simulink model "car_dynamics_sim"  (R2019b)
settings: Solver=VariableStepAuto  StartTime=0.0  StopTime=100  RelTol=1e-3
values from neighbouring files (symbols this model uses):
  air_density = 1.225    [main.m]
  drag_coefficient = 0.33    [main.m]
  equ_mass_of_rot_parts = (1/wheel_radius^2)*(wheel_inertia+motor_rotor_inertia*gearbox_ratio^2)    (= 15.059687787)    [main.m]
  gravity = 9.8    [main.m]
  mass = 900    [main.m]
  rolling_resistance_coefficient_0 = 0    [main.m]
  rolling_resistance_coefficient_1 = 0.01    [main.m]
  slope_of_track = 3    [main.m]
  surface_area = 2.14    [main.m]
  torque = 150    [main.m]
  wheel_radius = 0.165    [main.m]
undefined symbols (not defined in the file or in its folder): simulation_length_track
settings Model: Creator=jamil  LastModifiedBy=jamil

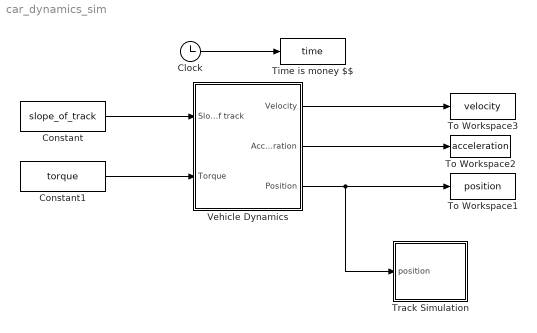
== system car_dynamics_sim ==
  Clock : Clock
  Constant : Constant  Value=slope_of_track
  Constant1 : Constant  Value=torque
  Time is money $$ : ToWorkspace  VariableName=time  SampleTime=-1
  To Workspace1 : ToWorkspace  VariableName=position  SampleTime=-1
  To Workspace2 : ToWorkspace  VariableName=acceleration  SampleTime=-1
  To Workspace3 : ToWorkspace  VariableName=velocity  SampleTime=-1
  Track Simulation : Subsystem
  Vehicle Dynamics : Subsystem
  wires:
  Constant/1 -> Vehicle Dynamics/1("Slope of track ")
  Constant1/1 -> Vehicle Dynamics/2(Torque)
  Vehicle Dynamics/1(Velocity) -> To Workspace3/1
  Vehicle Dynamics/2(Acceleration) -> To Workspace2/1
  Clock/1 -> Time is money $$/1
  Vehicle Dynamics/3(Position) -> Track Simulation/1(position), To Workspace1/1

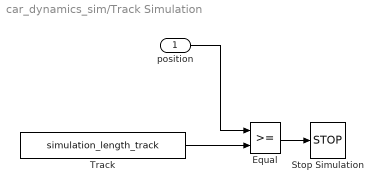
== system car_dynamics_sim/Track Simulation ==
  position : Inport
  Equal : RelationalOperator  OutDataTypeStr=boolean  RndMeth=Simplest
  Stop Simulation : Stop
  "Track " : Constant  Value=simulation_length_track
  wires:
  Equal/1 -> Stop Simulation/1
  position/1 -> Equal/1
  "Track "/1 -> Equal/2

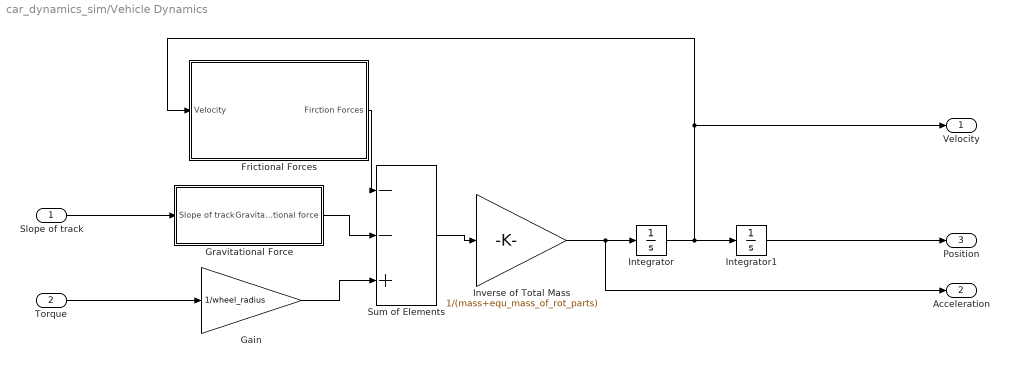
== system car_dynamics_sim/Vehicle Dynamics ==
  "Slope of track " : Inport
  Torque : Inport  Port=2
  Frictional Forces : Subsystem
  Gain : Gain  Gain=1/wheel_radius
  Gravitational Force : Subsystem
  Integrator : Integrator
  Integrator1 : Integrator
  Inverse of Total Mass : Gain  Gain=1/(mass+equ_mass_of_rot_parts)
  Sum of Elements : Sum  Inputs=--+
  Velocity : Outport
  Acceleration : Outport  Port=2
  Position : Outport  Port=3
  wires:
  Integrator/1 -> Integrator1/1, Frictional Forces/1(Velocity), Velocity/1
  Integrator1/1 -> Position/1
  Inverse of Total Mass/1 -> Acceleration/1, Integrator/1
  Sum of Elements/1 -> Inverse of Total Mass/1
  Frictional Forces/1(Firction Forces) -> Sum of Elements/1
  "Slope of track "/1 -> Gravitational Force/1(Slope of track)
  Gravitational Force/1(Gravitational force) -> Sum of Elements/2
  Torque/1 -> Gain/1
  Gain/1 -> Sum of Elements/3

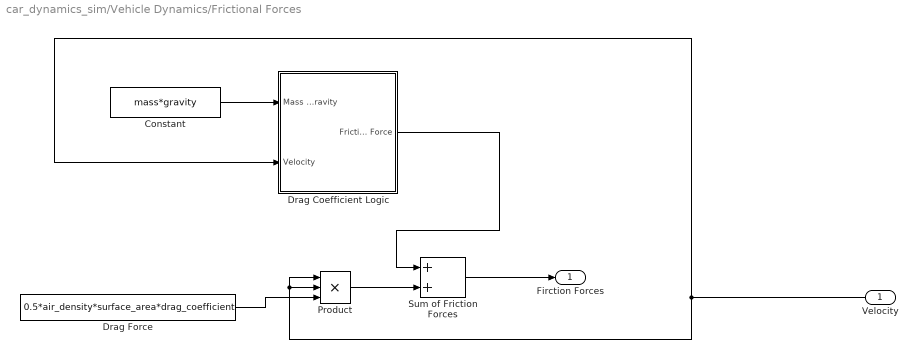
== system car_dynamics_sim/Vehicle Dynamics/Frictional Forces ==
  Velocity : Inport
  Constant : Constant  Value=mass*gravity
  Drag Coefficient Logic : Subsystem
  Drag Force : Constant  Value=0.5*air_density*surface_area*drag_coefficient
  Product : Product  Inputs=3
  Sum of Friction Forces : Sum
  Firction Forces : Outport
  wires:
  Sum of Friction Forces/1 -> Firction Forces/1
  Drag Force/1 -> Product/3
  Constant/1 -> Drag Coefficient Logic/1("Mass and Gravity ")
  Drag Coefficient Logic/1(Friction Force) -> Sum of Friction Forces/1
  Velocity/1 -> Drag Coefficient Logic/2(Velocity), Product/1, Product/2
  Product/1 -> Sum of Friction Forces/2

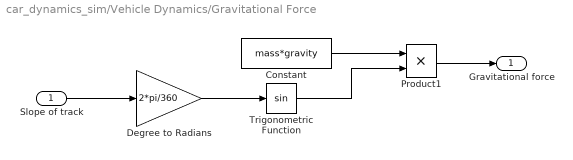
== system car_dynamics_sim/Vehicle Dynamics/Gravitational Force ==
  Slope of track : Inport
  Constant : Constant  Value=mass*gravity
  Degree to Radians : Gain  Gain=2*pi/360
  Product1 : Product
  Trigonometric Function : Trigonometry
  Gravitational force : Outport
  wires:
  Product1/1 -> Gravitational force/1
  Constant/1 -> Product1/1
  Trigonometric Function/1 -> Product1/2
  Slope of track/1 -> Degree to Radians/1
  Degree to Radians/1 -> Trigonometric Function/1

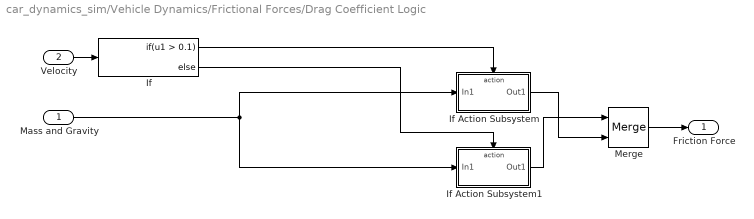
== system car_dynamics_sim/Vehicle Dynamics/Frictional Forces/Drag Coefficient Logic ==
  "Mass and Gravity " : Inport
  Velocity : Inport  Port=2
  If : If  IfExpression=u1 > 0.1
  If Action Subsystem : Subsystem  TreatAsAtomicUnit=on
  If Action Subsystem1 : Subsystem  TreatAsAtomicUnit=on
  Merge : Merge
  Friction Force : Outport
  wires:
  If Action Subsystem/1(Out1) -> Merge/2
  If Action Subsystem1/1(Out1) -> Merge/1
  If/2 -> If Action Subsystem1/Action
  "Mass and Gravity "/1 -> If Action Subsystem/1(In1), If Action Subsystem1/1(In1)
  Merge/1 -> Friction Force/1
  If/1 -> If Action Subsystem/Action
  Velocity/1 -> If/1

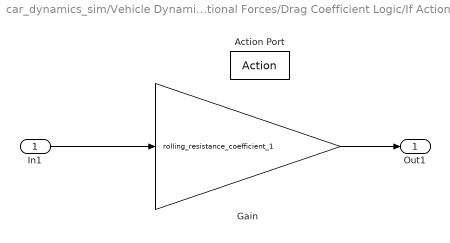
== system car_dynamics_sim/Vehicle Dynamics/Frictional Forces/Drag Coefficient Logic/If Action Subsystem ==
  In1 : Inport
  Action Port : ActionPort  ActionPortLabel=if(u1 > 0.1)
  Gain : Gain  Gain=rolling_resistance_coefficient_1
  Out1 : Outport
  wires:
  In1/1 -> Gain/1
  Gain/1 -> Out1/1

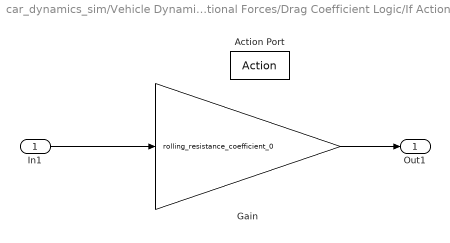
== system car_dynamics_sim/Vehicle Dynamics/Frictional Forces/Drag Coefficient Logic/If Action Subsystem1 ==
  In1 : Inport
  Action Port : ActionPort  ActionPortLabel=else
  Gain : Gain  Gain=rolling_resistance_coefficient_0
  Out1 : Outport
  wires:
  In1/1 -> Gain/1
  Gain/1 -> Out1/1
